simulink model "Sistema_tx_rx"  (R2024b)
settings: Solver=VariableStepAuto  StartTime=0.0  StopTime=0.005  RelTol=1e-3
undefined symbols (not defined in the file): Ts
libraries: dspsrcs4 x6, dspfdesign x3, commanapbnd3 x2
settings Model: Creator=river  LastModifiedBy=romaf41

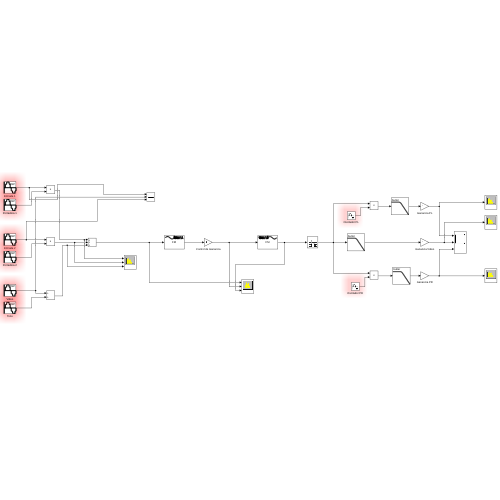
[thumbnail: Simulink's stored preview of the top-level diagram]
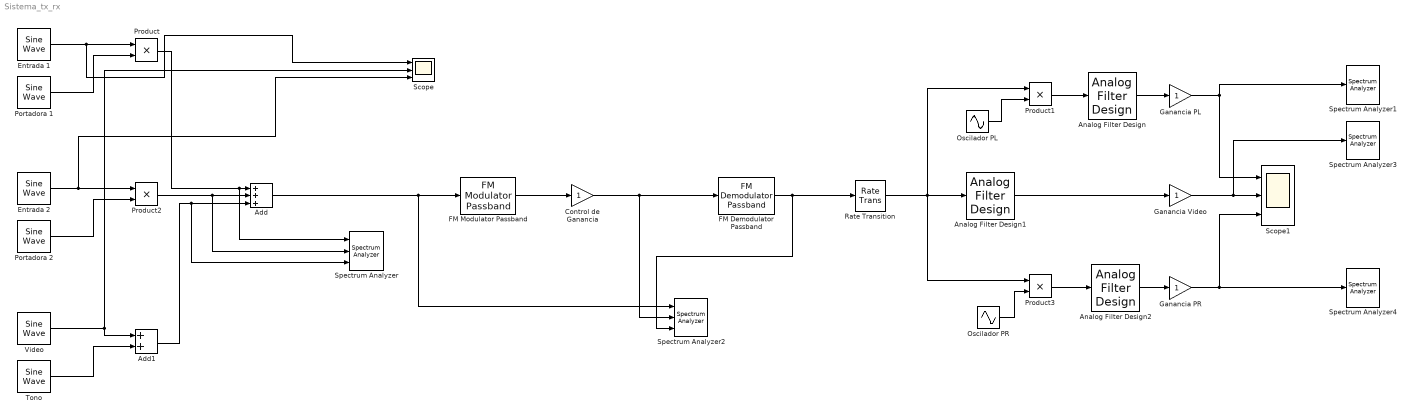
== system Sistema_tx_rx ==
  Add : Sum  Inputs=+++
  Add1 : Sum
  Analog Filter Design : dspfdesign/Analog Filter Design  method=Butterworth  filttype=Lowpass  N=5  Wlo=2*pi*16e3  Whi=2*pi*16e3  Rp=2  Rs=40
  Analog Filter Design1 : dspfdesign/Analog Filter Design  method=Butterworth  filttype=Lowpass  N=5  Wlo=2*pi*4.25e6  Whi=3200  Rp=2  Rs=40
  Analog Filter Design2 : dspfdesign/Analog Filter Design  method=Butterworth  filttype=Lowpass  N=5  Wlo=2*pi*16e3  Whi=2*pi*16e3  Rp=2  Rs=40
  Control de Ganancia : Gain
  Entrada 1 : dspsrcs4/Sine Wave  Amplitude=1  Frequency=15e3  Phase=0  SampleMode=Discrete  OutComplex=Real  CompMethod=Trigonometric fcn  TableSize=Speed  SampleTime=Ts  SamplesPerFrame=1  ResetState=Restart at time zero  OutputFrames=off  dataType=double  wordLen=16  udDataType=sfix(16)  fracBitsMode=Best precision  numFracBits=15  OutDataTypeStr=double  LastOutDataTypeStr=double
  Entrada 2 : dspsrcs4/Sine Wave  Amplitude=1  Frequency=15e3  Phase=0  SampleMode=Discrete  OutComplex=Real  CompMethod=Trigonometric fcn  TableSize=Speed  SampleTime=Ts  SamplesPerFrame=1  ResetState=Restart at time zero  OutputFrames=off  dataType=double  wordLen=16  udDataType=sfix(16)  fracBitsMode=Best precision  numFracBits=15  OutDataTypeStr=double  LastOutDataTypeStr=double
  FM Demodulator Passband : commanapbnd3/FM Demodulator Passband  Fc=400e6  Ph=0  Kc=2.5e6  Ho=100
  FM Modulator Passband : commanapbnd3/FM Modulator Passband  Fc=400e6  Ph=0  Kc=2.5e6
  Ganancia PL : Gain
  Ganancia PR : Gain
  Ganancia Video : Gain
  Oscilador PL : Sin  Frequency=2*pi*4.8e6  SampleTime=Ts
  Oscilador PR : Sin  Frequency=2*pi*5e6  SampleTime=Ts
  Portadora 1 : dspsrcs4/Sine Wave  Amplitude=1  Frequency=4.8e6  Phase=0  SampleMode=Discrete  OutComplex=Real  CompMethod=Trigonometric fcn  TableSize=Speed  SampleTime=Ts  SamplesPerFrame=1  ResetState=Restart at time zero  OutputFrames=off  dataType=double  wordLen=16  udDataType=sfix(16)  fracBitsMode=Best precision  numFracBits=15  OutDataTypeStr=double  LastOutDataTypeStr=double
  Portadora 2 : dspsrcs4/Sine Wave  Amplitude=1  Frequency=5e6  Phase=0  SampleMode=Discrete  OutComplex=Real  CompMethod=Trigonometric fcn  TableSize=Speed  SampleTime=Ts  SamplesPerFrame=1  ResetState=Restart at time zero  OutputFrames=off  dataType=double  wordLen=16  udDataType=sfix(16)  fracBitsMode=Best precision  numFracBits=15  OutDataTypeStr=double  LastOutDataTypeStr=double
  Product{,1..3} (4 alike) : Product
  Rate Transition : RateTransition
  Scope : Scope  NumInputPorts=3
  Scope1 : Scope  NumInputPorts=3
  Spectrum Analyzer : SpectrumAnalyzer  NumInputPorts=3  WindowPosition=[1081.000000,521.000000,960.000000,1043.000000,]  ScopeFrameLocation=window  RBWSource=Property  RBW=100000  Span=5849645.520984195  StartFrequency=-2924822.7604920976  StopFrequency=2924822.7604920976  VBWSource=Property  VBW=1000  YLimits=[-127.69085571,40.818986]  ShowLegend=on
  Spectrum Analyzer1 : SpectrumAnalyzer  WindowPosition=[3001.000000,521.000000,960.000000,1043.000000,]  ScopeFrameLocation=window  RBWSource=Property  RBW=100000  Span=5849645.520984195  StartFrequency=-2924822.7604920976  StopFrequency=2924822.7604920976  VBWSource=Property  VBW=1000  YLimits=[-121.1260528,40.19092513]  ShowLegend=on
  Spectrum Analyzer2 : SpectrumAnalyzer  NumInputPorts=3  WindowPosition=[2041.000000,521.000000,960.000000,1043.000000,]  ScopeFrameLocation=window  RBWSource=Property  RBW=100000  Span=5849645.520984195  StartFrequency=-2924822.7604920976  StopFrequency=2924822.7604920976  VBWSource=Property  VBW=1000  YLimits=[-121.1260528,40.19092513]  ShowLegend=on  SelectedToolstripTab=spectrumAnalyzerToolstrip.estimationTab
  Spectrum Analyzer3 : SpectrumAnalyzer  WindowPosition=[2041.000000,521.000000,960.000000,1043.000000,]  ScopeFrameLocation=window  RBWSource=Property  RBW=100000  Span=5849645.520984195  StartFrequency=-2924822.7604920976  StopFrequency=2924822.7604920976  VBWSource=Property  VBW=1000  YLimits=[-121.1260528,40.19092513]  ShowLegend=on
  Spectrum Analyzer4 : SpectrumAnalyzer  WindowPosition=[2041.000000,521.000000,960.000000,1043.000000,]  ScopeFrameLocation=window  RBWSource=Property  RBW=100000  Span=5849645.520984195  StartFrequency=-2924822.7604920976  StopFrequency=2924822.7604920976  VBWSource=Property  VBW=1000  YLimits=[-121.1260528,40.19092513]  ShowLegend=on
  Tono : dspsrcs4/Sine Wave  Amplitude=1  Frequency=4.5e6  Phase=0  SampleMode=Discrete  OutComplex=Real  CompMethod=Trigonometric fcn  TableSize=Speed  SampleTime=Ts  SamplesPerFrame=1  ResetState=Restart at time zero  OutputFrames=off  dataType=double  wordLen=16  udDataType=sfix(16)  fracBitsMode=Best precision  numFracBits=15  OutDataTypeStr=double  LastOutDataTypeStr=double
  Video : dspsrcs4/Sine Wave  Amplitude=1  Frequency=4.2e6  Phase=0  SampleMode=Discrete  OutComplex=Real  CompMethod=Trigonometric fcn  TableSize=Speed  SampleTime=Ts  SamplesPerFrame=1  ResetState=Restart at time zero  OutputFrames=off  dataType=double  wordLen=16  udDataType=sfix(16)  fracBitsMode=Best precision  numFracBits=15  OutDataTypeStr=double  LastOutDataTypeStr=double
  wires:
  Product2/1 -> Spectrum Analyzer/2, Add/2
  Add1/1 -> Spectrum Analyzer/3, Add/3
  Product/1 -> Spectrum Analyzer/1, Add/1
  Portadora 1/1 -> Product/2
  Portadora 2/1 -> Product2/2
  Video/1 -> Add1/1, Scope/2
  Tono/1 -> Add1/2
  Entrada 1/1 -> Scope/1, Product/1
  Entrada 2/1 -> Scope/3, Product2/1
  Add/1 -> Spectrum Analyzer2/1, FM Modulator Passband/1
  Analog Filter Design1/1 -> Ganancia Video/1
  Oscilador PR/1 -> Product3/2
  Product3/1 -> Analog Filter Design2/1
  Analog Filter Design2/1 -> Ganancia PR/1
  Ganancia Video/1 -> Spectrum Analyzer3/1, Scope1/2
  Ganancia PR/1 -> Spectrum Analyzer4/1, Scope1/3
  FM Modulator Passband/1 -> Control de Ganancia/1
  FM Demodulator Passband/1 -> Rate Transition/1, Spectrum Analyzer2/3
  Rate Transition/1 -> Product1/1, Product3/1, Analog Filter Design1/1
  Product1/1 -> Analog Filter Design/1
  Oscilador PL/1 -> Product1/2
  Ganancia PL/1 -> Scope1/1, Spectrum Analyzer1/1
  Analog Filter Design/1 -> Ganancia PL/1
  Control de Ganancia/1 -> FM Demodulator Passband/1, Spectrum Analyzer2/2
